simulink library "oceanForceCalculator_ul"  (R2018b)
settings: Solver=VariableStepAuto  StartTime=0.0  StopTime=10.0  RelTol=1e-3
values from neighbouring files (symbols this model uses):
  D = sum(normalVecMat'.*relVelGnd',2)    [oceanForceFunct.m]
  env = ENV.env    [groundStation001_ts2.m]    (also in groundStation001_ts3.m)
  gndStn = OCT.sixDoFStation    [groundStation001_ts3.m]
libraries: sharedutil x2, dspmtrx3 x1
settings Model: Creator=jcreed2  LastModifiedBy=jcreed2

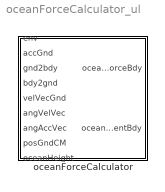
== system oceanForceCalculator_ul ==
  oceanForceCalculator : Subsystem  mask{Cdx=gndStn.cdX.Value, Cdy=gndStn.cdY.Value, Cdz=gndStn.cdZ.Value, Cax=gndStn.aMX.Value, Cay=gndStn.aMY.Value, Caz=gndStn.aMZ.Value, V=gndStn.volume.Value/(numel(gndStn.lumpedMassPositionMatrixBdy.Value)/3)}
      mask prompts: Cdx "Drag Coefficant x"; Cdy "Drag Coefficant y"; Cdz "Drag Coefficant z"; Cax "Added Mass Coefficant x"; Cay "Added Mass Coefficant y"; Caz "Added Mass Coefficant z"; V "Lumped Mass Volume"

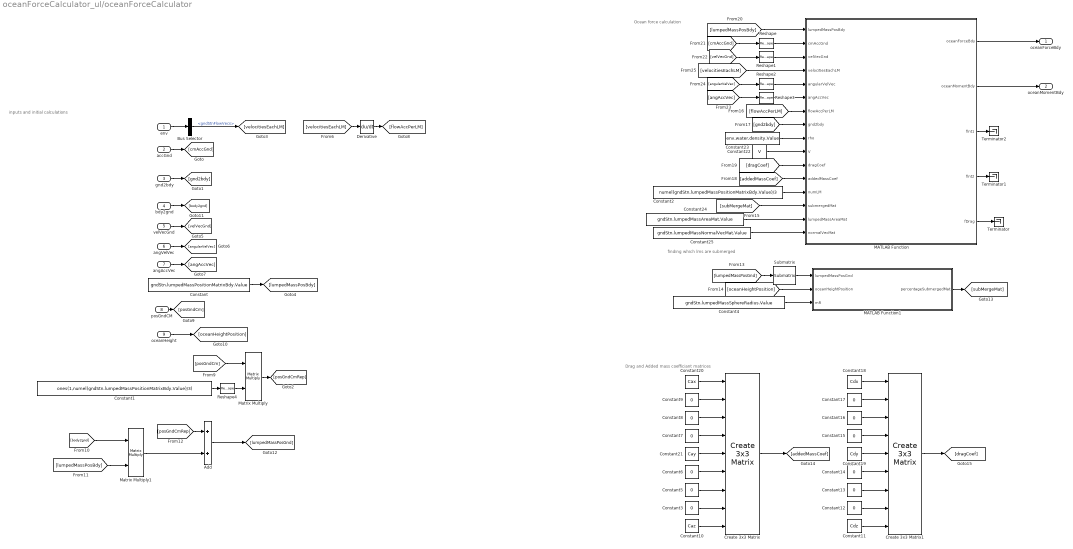
== system oceanForceCalculator_ul/oceanForceCalculator ==
  note: inputs and initial calculations
  note: Ocean force calculation
  note: finding which lms are submerged
  note: Drag and Added mass coefficiant matrices
  env : Inport
  accGnd : Inport  Port=2
  gnd2bdy : Inport  Port=3
  bdy2gnd : Inport  Port=4
  velVecGnd : Inport  Port=5
  angVelVec : Inport  Port=6
  angAccVec : Inport  Port=7
  posGndCM : Inport  Port=8
  oceanHeight : Inport  Port=9
  Add : Sum
  Bus Selector : BusSelector  OutputSignals=gndStnFlowVecs
  Constant : Constant  Value=gndStn.lumpedMassPositionMatrixBdy.Value
  Constant1 : Constant  Value=ones(1,numel(gndStn.lumpedMassPositionMatrixBdy.Value)/3)
  Constant10 : Constant  Value=Caz
  Constant11 : Constant  Value=Cdz
  Constant{3,5..9,12..17} (12 alike) : Constant  Value=0
  Constant18 : Constant  Value=Cdx
  Constant19 : Constant  Value=Cdy
  Constant2 : Constant  Value=numel(gndStn.lumpedMassPositionMatrixBdy.Value)/3
  Constant20 : Constant  Value=Cax
  Constant21 : Constant  Value=Cay
  Constant22 : Constant  Value=V
  Constant23 : Constant  Value=env.water.density.Value
  Constant24 : Constant  Value=gndStn.lumpedMassAreaMat.Value
  Constant25 : Constant  Value=gndStn.lumpedMassNormalVecMat.Value
  Constant4 : Constant  Value=gndStn.lumpedMassSphereRadius.Value
  Create 3x3 Matrix : sharedutil/Create 3x3 Matrix  aMode=aMode
  Create 3x3 Matrix1 : sharedutil/Create 3x3 Matrix  aMode=aMode
  Derivative : Derivative
  MATLAB Function : MATLAB Function  TreatAsAtomicUnit=on
  MATLAB Function1 : MATLAB Function  TreatAsAtomicUnit=on
  Matrix Multiply : Product  Multiplication=Matrix(*)
  Matrix Multiply1 : Product  Multiplication=Matrix(*)
  Reshape{,1..3} (4 alike) : Reshape  OutputDimensionality=Column vector (2-D)
  Reshape4 : Reshape  OutputDimensionality=Row vector (2-D)
  Submatrix : dspmtrx3/Submatrix  RowSpan=One row  RowStartMode=Last  RowStartIndex=1  RowEndMode=Last  RowEndIndex=1  ColSpan=All columns  ColStartMode=First  ColStartIndex=1  ColEndMode=Last  ColEndIndex=1
  Terminator : Terminator
  Terminator1 : Terminator
  Terminator2 : Terminator
  oceanForceBdy : Outport
  oceanMomentBdy : Outport  Port=2
  wires:
  Derivative/1 -> [flowAccPerLM]
  [velocitiesEachLM] -> Derivative/1
  angAccVec/1 -> [angAccVec]
  angVelVec/1 -> [angularVelVec]
  velVecGnd/1 -> [velVecGnd]
  Bus Selector/1 -> [velocitiesEachLM]  "<gndStnFlowVecs>"
  bdy2gnd/1 -> [body2gnd]
  gnd2bdy/1 -> [gnd2bdy]
  accGnd/1 -> [cmAccGnd]
  env/1 -> Bus Selector/1
  Constant/1 -> [lumpedMassPosBdy]
  Reshape/1 -> MATLAB Function/2(cmAccGnd)
  Reshape1/1 -> MATLAB Function/3(velVecGnd)
  Reshape2/1 -> MATLAB Function/5(angularVelVec)
  Reshape3/1 -> MATLAB Function/6(angAccVec)
  Reshape4/1 -> Matrix Multiply/2
  Matrix Multiply/1 -> [posGndCmRep]
  Constant1/1 -> Reshape4/1
  [posGndCm] -> Matrix Multiply/1
  posGndCM/1 -> [posGndCm]
  oceanHeight/1 -> [oceanHeightPosition]
  [body2gnd] -> Matrix Multiply1/1
  [lumpedMassPosBdy] -> Matrix Multiply1/2
  [posGndCmRep] -> Add/1
  Matrix Multiply1/1 -> Add/2
  Add/1 -> [lumpedMassPosGnd]
  [lumpedMassPosGnd] -> Submatrix/1
  [oceanHeightPosition] -> MATLAB Function1/2(oceanHeightPosition)
  Constant4/1 -> MATLAB Function1/3(mR)
  Submatrix/1 -> MATLAB Function1/1(lumpedMassPosGnd)
  MATLAB Function1/1(percentageSubmergedMat) -> [subMergeMat]
  [subMergeMat] -> MATLAB Function/14(submergedMat)
  [flowAccPerLM] -> MATLAB Function/7(flowAccPerLM)
  [gnd2bdy] -> MATLAB Function/8(gnd2bdy)
  Constant9/1 -> Create 3x3 Matrix/2
  Constant17/1 -> Create 3x3 Matrix1/2
  Constant8/1 -> Create 3x3 Matrix/3
  Constant12/1 -> Create 3x3 Matrix1/8
  Constant16/1 -> Create 3x3 Matrix1/3
  Create 3x3 Matrix1/1 -> [dragCoef]
  Constant14/1 -> Create 3x3 Matrix1/6
  Constant7/1 -> Create 3x3 Matrix/4
  Constant6/1 -> Create 3x3 Matrix/6
  Constant19/1 -> Create 3x3 Matrix1/5
  Constant21/1 -> Create 3x3 Matrix/5
  Constant20/1 -> Create 3x3 Matrix/1
  Constant18/1 -> Create 3x3 Matrix1/1
  Constant13/1 -> Create 3x3 Matrix1/7
  Constant10/1 -> Create 3x3 Matrix/9
  Constant3/1 -> Create 3x3 Matrix/8
  Constant5/1 -> Create 3x3 Matrix/7
  Constant11/1 -> Create 3x3 Matrix1/9
  Create 3x3 Matrix/1 -> [addedMassCoef]
  Constant15/1 -> Create 3x3 Matrix1/4
  [addedMassCoef] -> MATLAB Function/12(addedMassCoef)
  [dragCoef] -> MATLAB Function/11(dragCoef)
  Constant22/1 -> MATLAB Function/10(V)
  Constant23/1 -> MATLAB Function/9(rho)
  [lumpedMassPosBdy] -> MATLAB Function/1(lumpedMassPosBdy)
  [cmAccGnd] -> Reshape/1
  [velVecGnd] -> Reshape1/1
  MATLAB Function/1(oceanForceBdy) -> oceanForceBdy/1
  MATLAB Function/2(oceanMomentBdy) -> oceanMomentBdy/1
  [angAccVec] -> Reshape3/1
  [angularVelVec] -> Reshape2/1
  [velocitiesEachLM] -> MATLAB Function/4(velocitiesEachLM)
  Constant2/1 -> MATLAB Function/13(numLM)
  Constant24/1 -> MATLAB Function/15(lumpedMassAreaMat)
  Constant25/1 -> MATLAB Function/16(normalVecMat)
  MATLAB Function/5(fDrag) -> Terminator/1
  MATLAB Function/4(fInt2) -> Terminator1/1
  MATLAB Function/3(fInt1) -> Terminator2/1

== matlab function oceanForceCalculator_ul/oceanForceCalculator/MATLAB Function1 ==
  data: lumpedMassPosGnd input; percentageSubmergedMat output; oceanHeightPosition input; mR input
function percentageSubmergedMat  = fcn(lumpedMassPosGnd,oceanHeightPosition,mR)

%lumped Mass pos gnd is 3 by number of lumped masses

sz = size(lumpedMassPosGnd);
percentageSubmergedMat = zeros(1,sz(2));
matCat = [];

for i = sz(2):-1:1
    
    dist2surf = oceanHeightPosition(i) - lumpedMassPosGnd(:,i);
   
    
    
    if dist2surf >= mR
        
        percentSub = 1;
    elseif dist2surf <= -mR
        
        percentSub = 0;
    else
        
        percentSub = .5*dist2surf + .5;
    end
    
    
    matCat = [matCat,percentSub];
end

percentageSubmergedMat = percentageSubmergedMat+matCat;
end

== matlab function oceanForceCalculator_ul/oceanForceCalculator/MATLAB Function ==
  data: lumpedMassPosBdy input; oceanForceBdy output; oceanMomentBdy output; cmAccGnd input; velVecGnd input; velocitiesEachLM input; angularVelVec input; angAccVec input; flowAccPerLM input; gnd2bdy input; rho input; V input; dragCoef input; addedMassCoef input; numLM input; submergedMat input; lumpedMassAreaMat input; normalVecMat input; fInt1 output; fInt2 output; fDrag output
function [oceanForceBdy,oceanMomentBdy,fInt1,fInt2,fDrag] = fcn(lumpedMassPosBdy,cmAccGnd,velVecGnd,velocitiesEachLM,angularVelVec,angAccVec,...
    flowAccPerLM,gnd2bdy,rho,V,dragCoef,addedMassCoef,numLM,submergedMat,lumpedMassAreaMat,normalVecMat)





% [oceanForceBdy,oceanMomentBdy] = oceanForceFunct(lumpedMassPosBdy,cmAccGnd,velVecGnd,velocitiesEachLM,...
%     angularVelVec,angAccVec,flowAccPerLM,gnd2bdy,rho,V,dragCoef,addedMassCoef,numLM,submergedMat,lumpedMassAreaMat,normalVecMat);
% end




%% creating rep mats for vectorizing code
angAccVecMat = repmat(angAccVec,1,numLM);
cmAccGndMat = repmat(cmAccGnd,1,numLM);
velVecGndMat = repmat(velVecGnd,1,numLM);
angularVelVecMat = repmat(angularVelVec,1,numLM);
submergedMatT = submergedMat';



%% acceleration of each lumped mass point in the body frame

angACrossR = cross(angAccVecMat,lumpedMassPosBdy);

coriolas = cross(angularVelVecMat, lumpedMassPosBdy); % not really coriolas, just an intermiadiate step to get omega squared R


omegaSqrdR = cross(angularVelVecMat,coriolas );

accLMGnd = cmAccGndMat + angACrossR + omegaSqrdR;


%% Relative accelerations
relVelGnd = velocitiesEachLM - velVecGndMat  ;
relAccGnd = flowAccPerLM - accLMGnd    ;




%% Areas drag

D = sum(normalVecMat'.*relVelGnd',2);
LMAMT = lumpedMassAreaMat'; % lumped mass area mat transposed
RVGT = relVelGnd'; % vel veg gnd mat transposed, Im not sure if indexing and then transposing messes it up so I am transposing before
Aproj = zeros(numLM,3);
Aproj(D>0,:) = LMAMT(D>0,:).*RVGT(D>0,:);
fDrag = repmat(.5*rho*(sqrt(sum(RVGT.*RVGT,2)))',3,1).*(dragCoef*Aproj');


oceanForceGnd = zeros(3,numLM);

%% F int 1
fInt1 = rho*V*flowAccPerLM;

%% F int 2
fInt2 = rho*V*(addedMassCoef *relAccGnd);

%only the elements that are underwater
oceanForceGnd(:,submergedMatT>0) = fInt1(:,submergedMatT>0) + fInt2(:,submergedMatT>0) + fDrag(:,submergedMatT>0);

oceanForceBdy = sum(gnd2bdy*oceanForceGnd,2);

oceanMomentBdy = sum(cross(lumpedMassPosBdy,gnd2bdy*oceanForceGnd),2);







end
